simulink model "radia_ih_sample"  (R2026a)
settings: Solver=FixedStepDiscrete  StopTime=2  FixedStep=0.050000000000000003
libraries: simulink x1
settings Model: Creator=Administrator  LastModifiedBy=Administrator

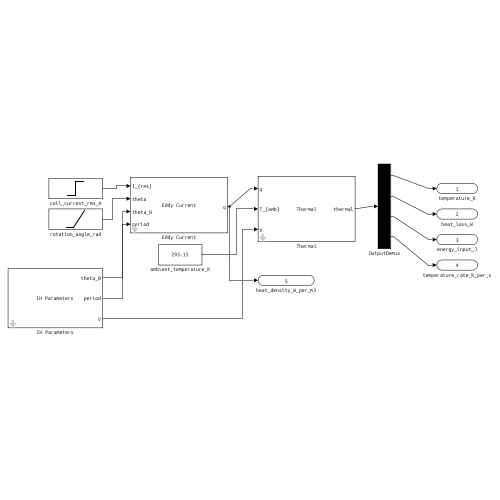
[thumbnail: Simulink's stored preview of the top-level diagram]
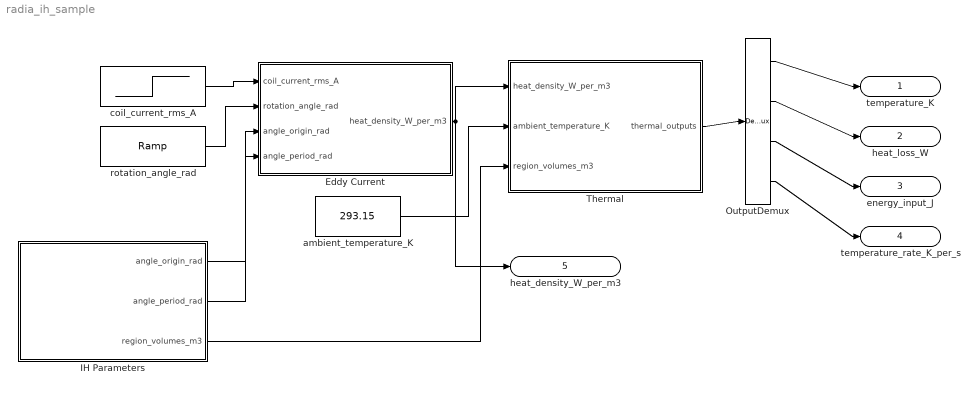
== system radia_ih_sample ==
  Eddy Current : Subsystem
      mask help: Periodic Radia heat-density map. At sample k it combines the current RMS carrier-current envelope with rotation angle k-1 and outputs one W/m^3 value per heated region.
      mask Display: disp('Eddy Current');port_label('input',1,'I_{rms}');port_label('input',2,'theta');port_label('input',3,'theta_0');port_label('input',4,'period');port_label('output',1,'q');
  IH Parameters : Subsystem  mask{angle_origin_rad=0, angle_period_rad=6.2831853071795862, region_volumes_m3=2.5000000000000001e-05, sample_time_s=0.050000000000000003, carrier_frequency_Hz=50000, thermal_backend=standard, region_names=workpiece}
      mask prompts: angle_origin_rad "Angle origin (rad)"; angle_period_rad "Angle period (rad)"; region_volumes_m3 "Region volumes (m^3)"; sample_time_s "Sample time (s)"; carrier_frequency_Hz "Carrier frequency (Hz)"; thermal_backend "Thermal backend"; region_names "Heated regions"
      mask help: Fixed IH model parameters. Current, rotation angle, and ambient temperature remain external Simulink signals.
      mask Display: disp('IH Parameters');port_label('output',1,'theta_0');port_label('output',2,'period');port_label('output',3,'V');
  OutputDemux : Demux
  Thermal : Subsystem
      mask help: Lumped thermal state model. Region heat densities are integrated over their volumes here; this subsystem alone owns temperature and energy state.
      mask Display: disp('Thermal');port_label('input',1,'q');port_label('input',2,'T_{amb}');port_label('input',3,'V');port_label('output',1,'thermal');
  ambient_temperature_K : Constant  Value=293.15
  coil_current_rms_A : Step  Time=0.5  InitialValue=40  FinalValue=80  SampleTime=0.05
  rotation_angle_rad : simulink/Sources/Ramp  slope=2*pi  start=0  InitialOutput=0
  temperature_K : Outport
  heat_loss_W : Outport  Port=2
  energy_input_J : Outport  Port=3
  temperature_rate_K_per_s : Outport  Port=4
  heat_density_W_per_m3 : Outport  Port=5
  wires:
  IH Parameters/1(angle_origin_rad) -> Eddy Current/3(angle_origin_rad)
  IH Parameters/2(angle_period_rad) -> Eddy Current/4(angle_period_rad)
  Eddy Current/1(heat_density_W_per_m3) -> Thermal/1(heat_density_W_per_m3), heat_density_W_per_m3/1
  IH Parameters/3(region_volumes_m3) -> Thermal/3(region_volumes_m3)
  Thermal/1(thermal_outputs) -> OutputDemux/1
  OutputDemux/1 -> temperature_K/1
  OutputDemux/2 -> heat_loss_W/1
  OutputDemux/3 -> energy_input_J/1
  OutputDemux/4 -> temperature_rate_K_per_s/1
  coil_current_rms_A/1 -> Eddy Current/1(coil_current_rms_A)
  rotation_angle_rad/1 -> Eddy Current/2(rotation_angle_rad)
  ambient_temperature_K/1 -> Thermal/2(ambient_temperature_K)

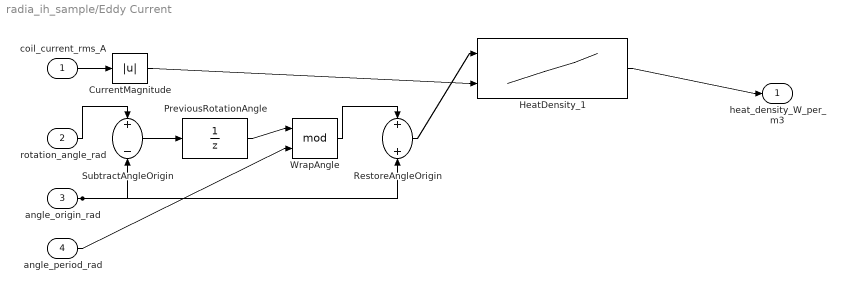
== system radia_ih_sample/Eddy Current ==
  coil_current_rms_A : Inport
  rotation_angle_rad : Inport  Port=2
  angle_origin_rad : Inport  Port=3
  angle_period_rad : Inport  Port=4
  CurrentMagnitude : Abs  SaturateOnIntegerOverflow=off
  HeatDensity_1 : Lookup_n-D  BreakpointsForDimension1=[0 1.5707963267948966 3.1415926535897931 4.7123889803846897 6.2831853071795862]  BreakpointsForDimension2=[0 50 100]  Table=[0 1000000 4000000;0 1200000 4800000;0 800000 3200000;0 1100000 4400000;0 1000000 4000000]  ExtrapMethod=Clip  InternalRulePriority=Speed  RndMeth=Simplest
      settings: InputPortMap=u0,u1
  PreviousRotationAngle : UnitDelay  SampleTime=0.050000000000000003
  RestoreAngleOrigin : Sum
  SubtractAngleOrigin : Sum  Inputs=+-
  WrapAngle : Math  Operator=mod
  heat_density_W_per_m3 : Outport
  wires:
  coil_current_rms_A/1 -> CurrentMagnitude/1
  rotation_angle_rad/1 -> SubtractAngleOrigin/1
  angle_origin_rad/1 -> SubtractAngleOrigin/2, RestoreAngleOrigin/2
  SubtractAngleOrigin/1 -> PreviousRotationAngle/1
  PreviousRotationAngle/1 -> WrapAngle/1
  angle_period_rad/1 -> WrapAngle/2
  WrapAngle/1 -> RestoreAngleOrigin/1
  RestoreAngleOrigin/1 -> HeatDensity_1/1
  CurrentMagnitude/1 -> HeatDensity_1/2
  HeatDensity_1/1 -> heat_density_W_per_m3/1

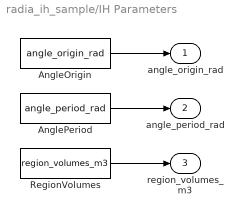
== system radia_ih_sample/IH Parameters ==
  AngleOrigin : Constant  Value=angle_origin_rad
  AnglePeriod : Constant  Value=angle_period_rad
  RegionVolumes : Constant  Value=region_volumes_m3
  angle_origin_rad : Outport
  angle_period_rad : Outport  Port=2
  region_volumes_m3 : Outport  Port=3
  wires:
  AngleOrigin/1 -> angle_origin_rad/1
  AnglePeriod/1 -> angle_period_rad/1
  RegionVolumes/1 -> region_volumes_m3/1

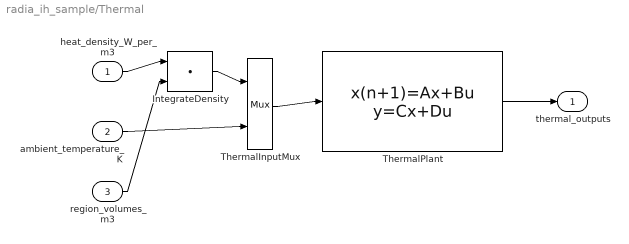
== system radia_ih_sample/Thermal ==
  heat_density_W_per_m3 : Inport
  ambient_temperature_K : Inport  Port=2
  region_volumes_m3 : Inport  Port=3
  IntegrateDensity : DotProduct  OutDataTypeStr=Inherit: Inherit via internal rule
  ThermalInputMux : Mux  Inputs=2
  ThermalPlant : DiscreteStateSpace  A=[0.99900049983337502 0;0 1]  B=[0.00033316672220832605 0.00099950016662497809;0.050000000000000003 0]  C=[1 0;3 0;0 1;-0.02 0]  D=[0 0;0 -3;0 0;0.0066666666666666671 0.02]  InitialCondition=[293.14999999999998;0]  SampleTime=0.050000000000000003
  thermal_outputs : Outport
  wires:
  heat_density_W_per_m3/1 -> IntegrateDensity/1
  region_volumes_m3/1 -> IntegrateDensity/2
  IntegrateDensity/1 -> ThermalInputMux/1
  ambient_temperature_K/1 -> ThermalInputMux/2
  ThermalInputMux/1 -> ThermalPlant/1
  ThermalPlant/1 -> thermal_outputs/1
